simulink model "OneDOF_PID"  (Simulink 9.1)
settings: Solver=VariableStepAuto  StartTime=0.0  StopTime=1000  RelTol=1e-3
values from neighbouring files (symbols this model uses):
  hd = 2    [OneDOF.m]    (also in PID_Controller.m = 100)
  hi = 10    [OneDOF.m]    (also in PID_Controller.m = 3)
  hp = 0.01    [OneDOF.m]    (also in PID_Controller.m = 0.001)
  kp = 6.32    [OneDOF.m]    (also in PID_Controller.m)
  mp = 0.16    [OneDOF.m]    (also in PID_Controller.m)
  omega_n = sqrt(kp/mp)    [OneDOF.m]    (also in PID_Controller.m)
settings Model: Creator=thomasperrein  LastModifiedBy=thomasperrein
settings DataIOCC: SaveFormat=Dataset  ReturnWorkspaceOutputs=on
settings OptimizationCC: LifeSpan=auto
settings DebuggingCC: UnderspecifiedInitializationDetection=Simplified  MergeDetectMultiDrivingBlocksExec=error  SFUnexpectedBacktrackingDiag=error  SFNoUnconditionalDefaultTransitionDiag=error  SFExecutionAtInitializationDiag=warning  SFMachineParentedDataDiag=error
settings HardwareCC: ProdBitPerPointer=64  ProdBitPerSizeT=64  ProdBitPerPtrDiffT=64  ProdLargestAtomicFloat=Float  ProdIntDivRoundTo=Zero  ProdEndianess=LittleEndian  ProdWordSize=64  ProdHWDeviceType=Intel->x86-64 (Windows64)
settings ModelReferenceCC: PropagateSignalLabelsOutOfModel=on
settings SFSimCC: SimUseLocalCustomCode=on
settings RTWCC: RTWUseLocalCustomCode=on
settings CodeAppCC: StateflowObjectComments=off
settings GRTTargetCC: TargetLangStandard=C99 (ISO)  CombineOutputUpdateFcns=on  GRTInterface=off
settings ConfigComp: CovMetricSettings=dwe  CovSaveCumulativeToWorkspaceVar=off  CovSaveSingleToWorkspaceVar=off  CovExternalEMLEnable=on

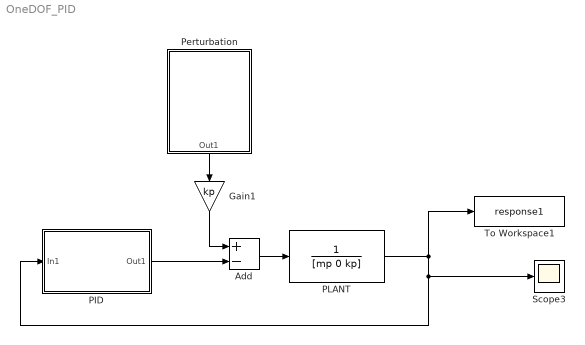
== system OneDOF_PID ==
  Add : Sum  Inputs=+-
  Gain1 : Gain  Gain=kp
  PID : Subsystem
  PLANT : TransferFcn  Denominator=[mp 0 kp]
  Perturbation : Subsystem
  Scope3 : Scope
  To Workspace1 : ToWorkspace  VariableName=response1  SaveFormat=Timeseries  SampleTime=-1
  wires:
  Perturbation/1(Out1) -> Gain1/1
  PID/1(Out1) -> Add/2
  Gain1/1 -> Add/1
  Add/1 -> PLANT/1
  PLANT/1 -> To Workspace1/1, Scope3/1, PID/1(In1)

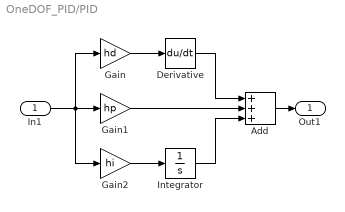
== system OneDOF_PID/PID ==
  In1 : Inport
  Add : Sum  Inputs=+++
  Derivative : Derivative
  Gain : Gain  Gain=hd
  Gain1 : Gain  Gain=hp
  Gain2 : Gain  Gain=hi
  Integrator : Integrator
  Out1 : Outport
  wires:
  Add/1 -> Out1/1
  Gain2/1 -> Integrator/1
  Gain1/1 -> Add/2
  Derivative/1 -> Add/1
  In1/1 -> Gain/1, Gain2/1, Gain1/1
  Gain/1 -> Derivative/1
  Integrator/1 -> Add/3

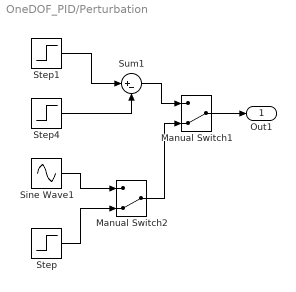
== system OneDOF_PID/Perturbation ==
  Manual Switch1 : ManualSwitch  CurrentSetting=0
  Manual Switch2 : ManualSwitch  CurrentSetting=0
  Sine Wave1 : Sin  Amplitude=0.05  Frequency=2*pi*omega_n  SampleTime=0
  Step : Step  Time=0  SampleTime=0
  Step1 : Step  Time=0  After=0.05  SampleTime=0
  Step4 : Step  Time=0.1  After=0.05  SampleTime=0
  Sum1 : Sum  Inputs=|+-
  Out1 : Outport
  wires:
  Manual Switch1/1 -> Out1/1
  Step4/1 -> Sum1/2
  Sum1/1 -> Manual Switch1/1
  Step1/1 -> Sum1/1
  Step/1 -> Manual Switch2/2
  Sine Wave1/1 -> Manual Switch2/1
  Manual Switch2/1 -> Manual Switch1/2
